simulink model "Adaptive_Simulation"  (R2018a)
settings: Solver=VariableStepAuto  StartTime=0.0  StopTime=100  RelTol=1e-3
values from neighbouring files (symbols this model uses):
  AT_filt_U = [0 1;-t2 -t1]    [Adaptive_Script.m]    (also in Non_Adaptive_Script.m)
  AT_filt_Y = [0 1;-t2 -t1]    [Adaptive_Script.m]    (also in Non_Adaptive_Script.m)
  Atheta = zeros(5,5)    [Adaptive_Script.m]
  BT_filt_U = [0;1]    [Adaptive_Script.m]    (also in Non_Adaptive_Script.m)
  BT_filt_Y = [0;1]    [Adaptive_Script.m]    (also in Non_Adaptive_Script.m)
  Btheta = -1*sign(Guessed_plant_Kp)*Gamma    [Adaptive_Script.m]
  CT_filt_U = [1 0; 0 1]    [Adaptive_Script.m]    (also in Non_Adaptive_Script.m = [G1(2) 0; 0 G1(1)])
  CT_filt_Y = [1 0; 0 1]    [Adaptive_Script.m]    (also in Non_Adaptive_Script.m = [F_bar(2) 0; 0 F_bar(1)])
  Ctheta = eye(5)    [Adaptive_Script.m]
  DT_filt_U = [0;0]    [Adaptive_Script.m]
  DT_filt_Y = [0;0]    [Adaptive_Script.m]
  Dtheta = zeros(5,5)    [Adaptive_Script.m]
  Ref_plant_Km = 1/time_const    (= 5)    [Adaptive_Script.m]    (also in Non_Adaptive_Script.m = 500)
  Ref_plant_Rm = [1 1/time_const]    [Adaptive_Script.m]    (also in Non_Adaptive_Script.m)
  True_plant_Kp = -0.5    [Adaptive_Script.m]    (also in Non_Adaptive_Script.m)
  True_plant_Rp = [1 0.4 4.3]    [Adaptive_Script.m]    (also in Non_Adaptive_Script.m)
  True_plant_Zp = [1 2]    [Adaptive_Script.m]    (also in Non_Adaptive_Script.m)
settings Model: Creator=ageng  LastModifiedBy=ageng

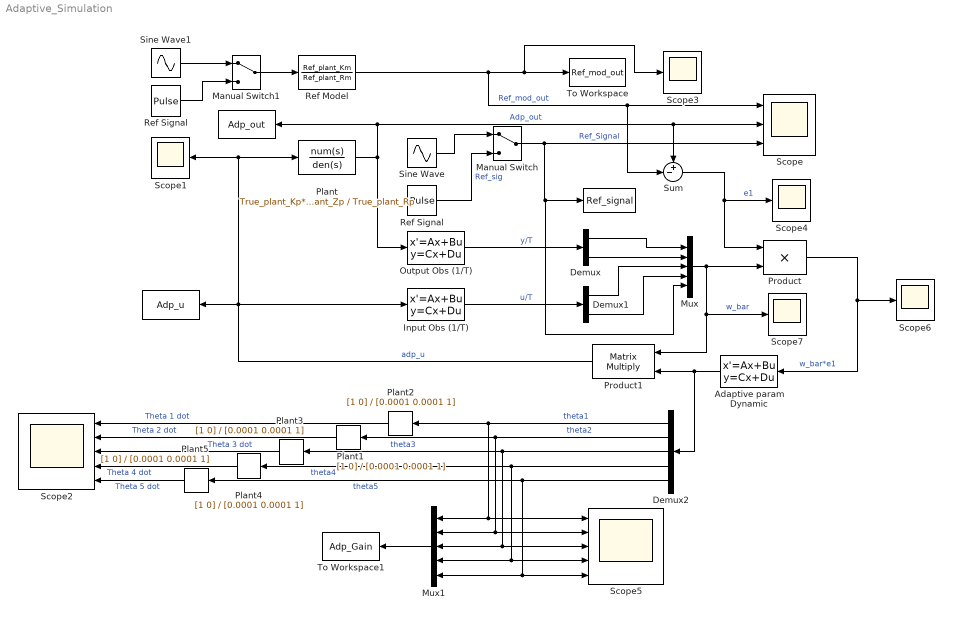
== system Adaptive_Simulation ==
  " " : ToWorkspace  VariableName=Adp_out  SaveFormat=Timeseries  SampleTime=0.001
      settings: Decimation=3
  "  " : ToWorkspace  VariableName=Ref_signal  SaveFormat=Timeseries  SampleTime=0.001
      settings: Decimation=3
  "     " : ToWorkspace  VariableName=Adp_u  SaveFormat=Timeseries  SampleTime=0.001
      settings: Decimation=3
  " Plant" : TransferFcn  Numerator=True_plant_Kp*True_plant_Zp  Denominator=True_plant_Rp
   Plant{1..5} (5 alike) : TransferFcn  Numerator=[1 0]  Denominator=[0.0001 0.0001 1]
  Adaptive param Dynamic : StateSpace  A=Atheta  B=Btheta  C=Ctheta  D=Dtheta  InitialCondition=Theta_init_bar'
  Demux : Demux  Outputs=2
  Demux1 : Demux  Outputs=2
  Demux2 : Demux  Outputs=5
  Input Obs (1/T) : StateSpace  A=AT_filt_U  B=BT_filt_U  C=CT_filt_U  D=DT_filt_U  InitialCondition=0
  Manual Switch : ManualSwitch
  Manual Switch1 : ManualSwitch
  Mux : Mux  Inputs=5
  Mux1 : Mux  Inputs=5
  Output Obs (1/T) : StateSpace  A=AT_filt_Y  B=BT_filt_Y  C=CT_filt_Y  D=DT_filt_Y  InitialCondition=0
  Product : Product
  Product1 : Product  Multiplication=Matrix(*)
  Ref Model : TransferFcn  Numerator=Ref_plant_Km  Denominator=Ref_plant_Rm
  Ref Signal : DiscretePulseGenerator  PulseType=Time based  Period=20  PulseWidth=50
  "Ref Signal " : DiscretePulseGenerator  PulseType=Time based  Period=20  PulseWidth=50
  Scope : Scope  NumInputPorts=3
  Scope{1,3..4,6..7} (5 alike) : Scope
  Scope2 : Scope  NumInputPorts=5
  Scope5 : Scope  NumInputPorts=5
  Sine Wave : Sin  Amplitude=10  Frequency=0.1  SampleTime=0
  Sine Wave1 : Sin  Amplitude=10  Frequency=0.1  SampleTime=0
  Sum : Sum  Inputs=+-|
  To Workspace : ToWorkspace  VariableName=Ref_mod_out  SaveFormat=Timeseries  SampleTime=0.001
      settings: Decimation=3
  To Workspace1 : ToWorkspace  VariableName=Adp_Gain  SaveFormat=Timeseries  SampleTime=0.0001
      settings: Decimation=2
  wires:
  " Plant"/1 -> " "/1, Sum/1, Scope/2, Output Obs (1/T)/1  "Adp_out"
  Output Obs (1/T)/1 -> Demux/1  "y/T"
  Input Obs (1/T)/1 -> Demux1/1  "u/T"
  Ref Signal/1 -> Manual Switch/2  "Ref_sig"
  Product1/1 -> " Plant"/1, Scope1/1, "     "/1, Input Obs (1/T)/1  "adp_u"
  "Ref Signal "/1 -> Manual Switch1/2
  Ref Model/1 -> Scope3/1, To Workspace/1, Sum/2, Scope/1  "Ref_mod_out"
  Sum/1 -> Scope4/1, Product/1  "e1"
  Mux/1 -> Scope7/1, Product1/1, Product/2  "w_bar"
  Product/1 -> Scope6/1, Adaptive param Dynamic/1  "w_bar*e1"
  Adaptive param Dynamic/1 -> Demux2/1, Product1/2
  Demux2/1 -> " Plant2"/1, Scope5/1, Mux1/1  "theta1"
  Demux2/2 -> " Plant1"/1, Mux1/2, Scope5/2  "theta2"
  Demux2/3 -> " Plant3"/1, Scope5/3, Mux1/3  "theta3"
  Demux2/4 -> " Plant4"/1, Scope5/4, Mux1/4  "theta4"
  Demux2/5 -> " Plant5"/1, Scope5/5, Mux1/5  "theta5"
  Mux1/1 -> To Workspace1/1
  Sine Wave/1 -> Manual Switch/1
  Manual Switch/1 -> Mux/5, "  "/1, Scope/3  "Ref_Signal"
  Sine Wave1/1 -> Manual Switch1/1
  Manual Switch1/1 -> Ref Model/1
  " Plant2"/1 -> Scope2/1  "Theta 1 dot"
  " Plant1"/1 -> Scope2/2  "Theta 2 dot"
  " Plant3"/1 -> Scope2/3  "Theta 3 dot"
  " Plant4"/1 -> Scope2/4  "Theta 4 dot"
  " Plant5"/1 -> Scope2/5  "Theta 5 dot"
  Demux/2 -> Mux/2
  Demux/1 -> Mux/1
  Demux1/1 -> Mux/3
  Demux1/2 -> Mux/4
